simulink model "Derivee_matrice_jacobienne"  (R2022b)
settings: Solver=VariableStepAuto  StartTime=0.0  StopTime=10.0  RelTol=1e-3
undefined symbols (not defined in the file): l1, l2
settings Model: Creator=cheye  LastModifiedBy=cheye

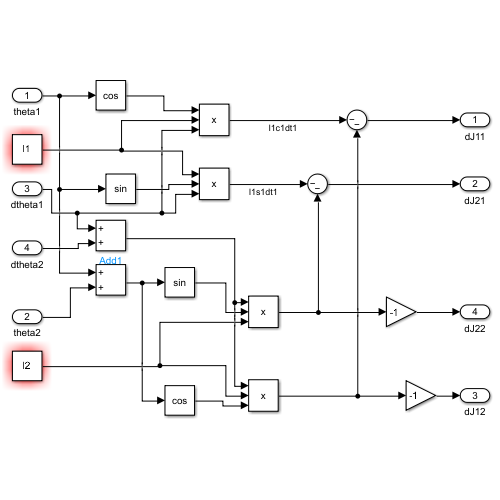
[thumbnail: Simulink's stored preview of the top-level diagram]
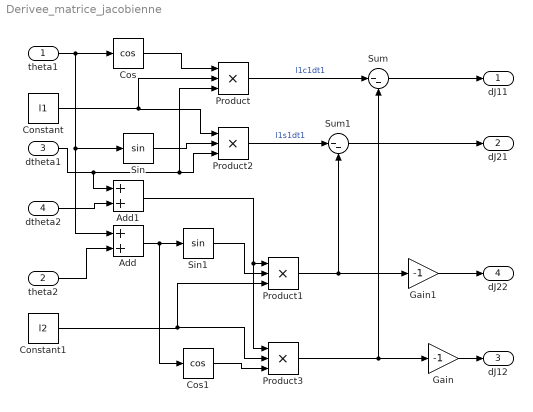
== system Derivee_matrice_jacobienne ==
  theta1 : Inport
  theta2 : Inport  Port=2
  dtheta1 : Inport  Port=3
  dtheta2 : Inport  Port=4
  Add : Sum
  Add1 : Sum
  Constant : Constant  Value=l1
  Constant1 : Constant  Value=l2
  Cos : Trigonometry  Operator=cos
  Cos1 : Trigonometry  Operator=cos
  Gain : Gain  Gain=-1
  Gain1 : Gain  Gain=-1
  Product{,1..3} (4 alike) : Product  Inputs=3
  Sin : Trigonometry
  Sin1 : Trigonometry
  Sum : Sum  Inputs=|--
  Sum1 : Sum  Inputs=|--
  dJ11 : Outport
  dJ21 : Outport  Port=2
  dJ12 : Outport  Port=3
  dJ22 : Outport  Port=4
  wires:
  Gain/1 -> dJ12/1
  Sum1/1 -> dJ21/1
  theta1/1 -> Cos/1, Sin/1, Add/1
  Product2/1 -> Sum1/1  "l1s1dt1"
  theta2/1 -> Add/2
  Constant1/1 -> Product3/2, Product1/3
  Sum/1 -> dJ11/1
  Sin1/1 -> Product1/2
  Cos/1 -> Product/1
  Cos1/1 -> Product3/3
  Add/1 -> Cos1/1, Sin1/1
  Constant/1 -> Product/2, Product2/1
  Product/1 -> Sum/1  "l1c1dt1"
  Sin/1 -> Product2/2
  dtheta1/1 -> Add1/1, Product/3, Product2/3
  Gain1/1 -> dJ22/1
  dtheta2/1 -> Add1/2
  Add1/1 -> Product3/1, Product1/1
  Product3/1 -> Sum/2, Gain/1
  Product1/1 -> Gain1/1, Sum1/2
